simulink model "dmpc"  (R2021a)
settings: Solver=ode4  StartTime=0.0  StopTime=10  FixedStep=simTs  RelTol=1e-3
values from neighbouring files (symbols this model uses):
  simTs = 1e-6    (= 1e-06)    [model.m]
  Ts = 80e-3    (= 0.08)    [model.m]
libraries: pid_lib x9, spsThreePhaseSeriesRLCBranchLib x9, spsabctodq0Lib x9, spsRMSLib x6, spsThreePhaseVIMeasurementLib x6, spsFirstOrderFilterLib x6, spsSecondOrderFilterLib x6, spsThreePhaseSeriesRLCLoadLib x4, spsFourierLib x3, spsPWMGenerator2LevelLib x3, spsdq0toabcLib x3, spsCurrentMeasurementLib x3
(part 1 of 2)
settings Model: SimulationMode=accelerator  Creator=Sameer Kumar  LastModifiedBy=Sameer Kumar

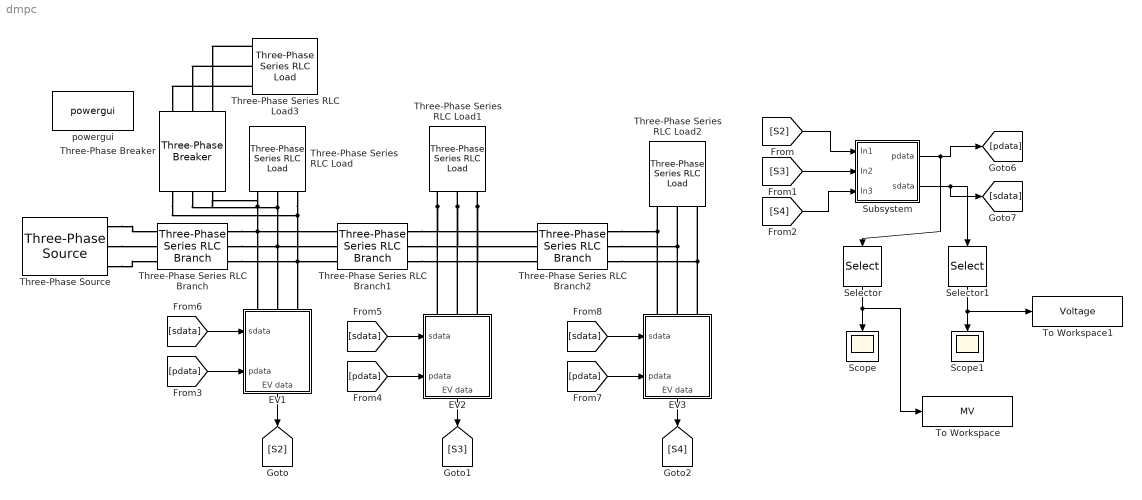
== system dmpc ==
  EV1 : Subsystem
      settings: PortSchema="{\"entries\":[{\"content\":{\"sides\":[{\"content\":{\"connectorIds\":[\"LConn1\",\"LConn2\",\"LConn3\"]},\"type\":\"ConnectorPlacement.EquallySpacedRectSide\",\"uuid\":\"b1121362-91a5-4336-a6ad-67b3009c2f66\"},{\"content\":{\"connectorIds\":[\"Out1\"],\"side\":\"RIGHT\"},\"type\":\"ConnectorPlacement.EquallySpacedRectSide\",\"uuid\":\"ba666203-56ee-4aa1-80fa-3bec4e81a32f\"},{\"content\":{\"connectorIds\":[\"In1\",\"In2\"],\"side\":\"TOP\"},\"type\":\"ConnectorPlacement.EquallySpacedRectSide\",\"uuid\":\"ec91c225-dc43-4f31-ad74-0ab1fa7bfdf2\"}]},\"type\":\"ConnectorPlacement.EquallySpacedConnector\",\"uuid\":\"9ad0d362-2acd-4c24-addb-fb01ea261cc5\"}],\"packageUris\":[\"http://schema.mathworks.com/mf0/Connector/R2020b\"],\"version\":\"1.0\"}"
  EV2 : Subsystem
      settings: PortSchema="{\"entries\":[{\"content\":{\"sides\":[{\"content\":{\"connectorIds\":[\"LConn1\",\"LConn2\",\"LConn3\"]},\"type\":\"ConnectorPlacement.EquallySpacedRectSide\",\"uuid\":\"b1121362-91a5-4336-a6ad-67b3009c2f66\"},{\"content\":{\"connectorIds\":[\"Out1\"],\"side\":\"RIGHT\"},\"type\":\"ConnectorPlacement.EquallySpacedRectSide\",\"uuid\":\"ba666203-56ee-4aa1-80fa-3bec4e81a32f\"},{\"content\":{\"connectorIds\":[\"In1\",\"In2\"],\"side\":\"TOP\"},\"type\":\"ConnectorPlacement.EquallySpacedRectSide\",\"uuid\":\"ec91c225-dc43-4f31-ad74-0ab1fa7bfdf2\"}]},\"type\":\"ConnectorPlacement.EquallySpacedConnector\",\"uuid\":\"9ad0d362-2acd-4c24-addb-fb01ea261cc5\"}],\"packageUris\":[\"http://schema.mathworks.com/mf0/Connector/R2020b\"],\"version\":\"1.0\"}"
  EV3 : Subsystem
      settings: PortSchema="{\"entries\":[{\"content\":{\"sides\":[{\"content\":{\"connectorIds\":[\"LConn1\",\"LConn2\",\"LConn3\"]},\"type\":\"ConnectorPlacement.EquallySpacedRectSide\",\"uuid\":\"b1121362-91a5-4336-a6ad-67b3009c2f66\"},{\"content\":{\"connectorIds\":[\"Out1\"],\"side\":\"RIGHT\"},\"type\":\"ConnectorPlacement.EquallySpacedRectSide\",\"uuid\":\"ba666203-56ee-4aa1-80fa-3bec4e81a32f\"},{\"content\":{\"connectorIds\":[\"In1\",\"In2\"],\"side\":\"TOP\"},\"type\":\"ConnectorPlacement.EquallySpacedRectSide\",\"uuid\":\"ec91c225-dc43-4f31-ad74-0ab1fa7bfdf2\"}]},\"type\":\"ConnectorPlacement.EquallySpacedConnector\",\"uuid\":\"9ad0d362-2acd-4c24-addb-fb01ea261cc5\"}],\"packageUris\":[\"http://schema.mathworks.com/mf0/Connector/R2020b\"],\"version\":\"1.0\"}"
  Scope : Scope
  Scope1 : Scope
  Selector : Selector  InputPortWidth=24  IndexOptions=Index vector (dialog)  Indices=[1 9 17]  OutputSizes=1
  Selector1 : Selector  InputPortWidth=8  IndexOptions=Index vector (dialog)  Indices=[6 7 8]  OutputSizes=1
  Subsystem : Subsystem
  Three-Phase Series RLC Branch : spsThreePhaseSeriesRLCBranchLib/Three-Phase Series RLC Branch  LConnTagsString=A|B|C  RConnTagsString=A|B|C  BranchType=RL  Resistance=0.05  Inductance=0.75e-3  Capacitance=1e-6  Measurements=None
  Three-Phase Series RLC Branch1 : spsThreePhaseSeriesRLCBranchLib/Three-Phase Series RLC Branch  LConnTagsString=A|B|C  RConnTagsString=A|B|C  BranchType=RL  Resistance=0.05  Inductance=0.15e-3  Capacitance=1e-6  Measurements=None
  Three-Phase Series RLC Branch2 : spsThreePhaseSeriesRLCBranchLib/Three-Phase Series RLC Branch  LConnTagsString=A|B|C  RConnTagsString=A|B|C  BranchType=RL  Resistance=0.05  Inductance=0.15e-3  Capacitance=1e-6  Measurements=None
  Three-Phase Series RLC Load : spsThreePhaseSeriesRLCLoadLib/Three-Phase Series RLC Load  LConnTagsString=A|B|C  Configuration=Y (grounded)  NominalVoltage=400  Vabc=[1e3 1e3 1e3]  Vabcp=[1e3 1e3 1e3]  NominalFrequency=50  UnbalancedPower=off  ActivePower=5e3  InductivePower=1.5e3  CapacitivePower=0  Pabc=[10e3 9e3 11e3]  QLabc=[100 90 110]  QCabc=[100 90 110]  Pabcp=[10e3 9e3 11e3]  QLabcp=[100 90 110]  QCabcp=[100 90 110]  Measurements=None  LoadType=constant Z
  Three-Phase Series RLC Load1 : spsThreePhaseSeriesRLCLoadLib/Three-Phase Series RLC Load  LConnTagsString=A|B|C  Configuration=Y (grounded)  NominalVoltage=400  Vabc=[1e3 1e3 1e3]  Vabcp=[1e3 1e3 1e3]  NominalFrequency=50  UnbalancedPower=off  ActivePower=5e3  InductivePower=1e3  CapacitivePower=0  Pabc=[10e3 9e3 11e3]  QLabc=[100 90 110]  QCabc=[100 90 110]  Pabcp=[10e3 9e3 11e3]  QLabcp=[100 90 110]  QCabcp=[100 90 110]  Measurements=None  LoadType=constant Z
  Three-Phase Series RLC Load2 : spsThreePhaseSeriesRLCLoadLib/Three-Phase Series RLC Load  LConnTagsString=A|B|C  Configuration=Y (grounded)  NominalVoltage=400  Vabc=[1e3 1e3 1e3]  Vabcp=[1e3 1e3 1e3]  NominalFrequency=50  UnbalancedPower=off  ActivePower=5e3  InductivePower=1e3  CapacitivePower=0  Pabc=[10e3 9e3 11e3]  QLabc=[100 90 110]  QCabc=[100 90 110]  Pabcp=[10e3 9e3 11e3]  QLabcp=[100 90 110]  QCabcp=[100 90 110]  Measurements=None  LoadType=constant Z
  Three-Phase Series RLC Load3 : spsThreePhaseSeriesRLCLoadLib/Three-Phase Series RLC Load  LConnTagsString=A|B|C  Configuration=Y (grounded)  NominalVoltage=400  Vabc=[1e3 1e3 1e3]  Vabcp=[1e3 1e3 1e3]  NominalFrequency=50  UnbalancedPower=off  ActivePower=0.1e-3  InductivePower=1.5e3  CapacitivePower=0  Pabc=[10e3 9e3 11e3]  QLabc=[100 90 110]  QCabc=[100 90 110]  Pabcp=[10e3 9e3 11e3]  QLabcp=[100 90 110]  QCabcp=[100 90 110]  Measurements=None  LoadType=constant Z
  Three-Phase Breaker : spsThreePhaseBreakerLib/Three-Phase Breaker  InitialState=open  SwitchA=on  SwitchB=on  SwitchC=on  SwitchTimes=[4]  External=off  BreakerResistance=1e-5  SnubberResistance=1e6  SnubberCapacitance=inf  Measurements=None
  Three-Phase Source : spsThreePhaseSourceLib/Three-Phase Source  InternalConnection=Yg  VoltagePhases=off  Voltage=400  PhaseAngle=0  Voltage_phases=[25e3 25e3 25e3]/sqrt(3)  PhaseAngles_phases=[0 -120 +120]  Frequency=50  NonIdealSource=on  SpecifyImpedance=off  Resistance=0  Inductance=0  ShortCircuitLevel=100e6  BaseVoltage=400  XRratio=7  BusType=swing  Pref=10e3  Qref=0  Prefabc=[10e3, 10e3, 10e3]  Qrefabc=[0, 0, 0]  Qmin=-inf  Qmax=inf
  To Workspace : ToWorkspace  VariableName=MV  SaveFormat=Timeseries  SampleTime=-1
  To Workspace1 : ToWorkspace  VariableName=Voltage  SaveFormat=Timeseries  SampleTime=-1
  powergui : spspowerguiLib/powergui  Priority=1  SimulationMode=Discrete  SampleTime=simTs  frequency=60  Iterations=50  frequencyindice=0  Pbase=100e6  ErrMax=1e-4  UnitsV=kV  UnitsW=MW  buscounter=0  FunctionMessages=off  echomessages=off  EnableUseOfTLC=off  CurrentSourceSwitches=off  DisableSnubberDevices=off  DisableRonSwitches=off  DisableVfSwitches=off  DisplayEquations=off  AutomaticDiscreteSolvers=off  SolverType=Tustin/Backward Euler (TBE)  Interpol=off  ExternalGateDelay=off  methode=off  Ts=100  x0status=blocks  SPID=on  SwTol=0  HookPort=off  NonlinearTolerance=1e-4  nMaxIteration=100  ContinueOnMaxIteration=off  RestoreLinks=warning  ResistiveCurrentMeasurement=off  Frange=[0:2:500]  Ylog=off  Xlog=on  ShowGrid=off  save=off  variable=ZData  structure=0  ZoomFFT=off  StartTime=0.0  cycles=1  DisplayStyle=1  fundamental=60  FreqAxis=off  MaxFrequency=1000  frequencyindicesteady=1  RmsSteady=1  display=off
  wires:
  [sdata] -> EV1/1(sdata)
  EV1/1(EV data) -> [S2]
  [pdata] -> EV1/2(pdata)
  [pdata] -> EV2/2(pdata)
  EV2/1(EV data) -> [S3]
  [sdata] -> EV2/1(sdata)
  [pdata] -> EV3/2(pdata)
  EV3/1(EV data) -> [S4]
  [sdata] -> EV3/1(sdata)
  [S2] -> Subsystem/1(In1)
  [S3] -> Subsystem/2(In2)
  [S4] -> Subsystem/3(In3)
  Subsystem/1(pdata) -> [pdata], Selector/1
  Subsystem/2(sdata) -> Selector1/1, [sdata]
  Selector/1 -> To Workspace/1, Scope/1
  Selector1/1 -> To Workspace1/1, Scope1/1
  connections:
  Three-Phase Series RLC Branch2/RConn3 -- EV3/LConn3 -- Three-Phase Series RLC Load2/LConn3
  Three-Phase Series RLC Load1/LConn3 -- EV2/LConn3 -- Three-Phase Series RLC Branch1/RConn3 -- Three-Phase Series RLC Branch2/LConn3
  Three-Phase Series RLC Branch2/RConn1 -- EV3/LConn1 -- Three-Phase Series RLC Load2/LConn1
  Three-Phase Series RLC Load/LConn1 -- Three-Phase Breaker/RConn1 -- EV1/LConn1 -- Three-Phase Series RLC Branch/RConn1 -- Three-Phase Series RLC Branch1/LConn1
  Three-Phase Series RLC Branch2/RConn2 -- EV3/LConn2 -- Three-Phase Series RLC Load2/LConn2
  Three-Phase Series RLC Load1/LConn2 -- EV2/LConn2 -- Three-Phase Series RLC Branch1/RConn2 -- Three-Phase Series RLC Branch2/LConn2
  Three-Phase Series RLC Load/LConn2 -- Three-Phase Breaker/RConn2 -- EV1/LConn2 -- Three-Phase Series RLC Branch1/LConn2 -- Three-Phase Series RLC Branch/RConn2
  Three-Phase Series RLC Load1/LConn1 -- EV2/LConn1 -- Three-Phase Series RLC Branch1/RConn1 -- Three-Phase Series RLC Branch2/LConn1
  Three-Phase Series RLC Load/LConn3 -- Three-Phase Breaker/RConn3 -- Three-Phase Series RLC Branch1/LConn3 -- EV1/LConn3 -- Three-Phase Series RLC Branch/RConn3
  Three-Phase Source/RConn3 -- Three-Phase Series RLC Branch/LConn3
  Three-Phase Source/RConn1 -- Three-Phase Series RLC Branch/LConn1
  Three-Phase Source/RConn2 -- Three-Phase Series RLC Branch/LConn2
  Three-Phase Series RLC Load3/LConn1 -- Three-Phase Breaker/LConn1
  Three-Phase Series RLC Load3/LConn2 -- Three-Phase Breaker/LConn2
  Three-Phase Series RLC Load3/LConn3 -- Three-Phase Breaker/LConn3

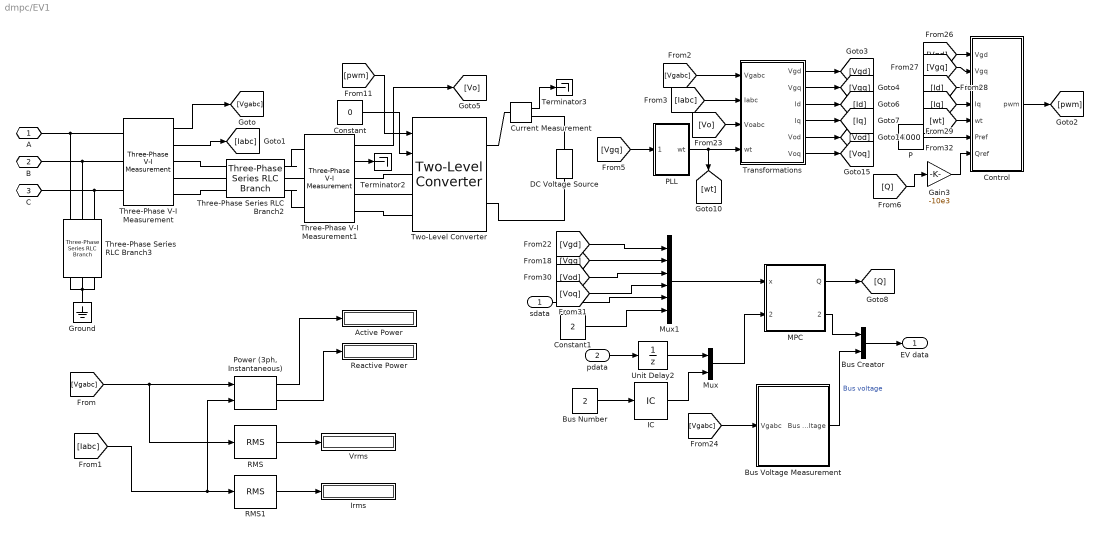
== system dmpc/EV1 ==
  sdata : Inport
  pdata : Inport  Port=2
  Active Power : Display
  Bus Creator : BusCreator  Inputs=2
  Bus Number : Constant  Value=2
  Bus Voltage Measurement : Subsystem
  Constant : Constant  Value=0
  Constant1 : Constant  Value=2
  Control : Subsystem
  Current Measurement : spsCurrentMeasurementLib/Current Measurement  PhasorSimulation=off  OutputType=Complex  PSBequivalent=0
  DC Voltage Source : spsDCVoltageSourceLib/DC Voltage Source  Amplitude=800  Measurements=None
  Gain3 : Gain  Gain=-10e3
  Ground : spsGroundLib/Ground  LConnTagsString=a
  IC : InitialCondition  Value=2
  Irms : Display
  MPC : Subsystem
  Mux : Mux  Inputs=2
  Mux1 : Mux  Inputs=6
  P : Constant  Value=6000
  PLL : Subsystem
  "Power (3ph, Instantaneous)" : spsPower3phInstantaneousLib/Power (3ph, Instantaneous)
  RMS : spsRMSLib/RMS  TrueRMS=on  Freq=50  RMSInit=220  Ts=simTs
  RMS1 : spsRMSLib/RMS  TrueRMS=on  Freq=50  RMSInit=10  Ts=simTs
  Reactive Power : Display
  Terminator2 : Terminator
  Terminator3 : Terminator
  Three-Phase Series RLC Branch2 : spsThreePhaseSeriesRLCBranchLib/Three-Phase Series RLC Branch  LConnTagsString=A|B|C  RConnTagsString=A|B|C  BranchType=RL  Resistance=0.1  Inductance=10e-3  Capacitance=1e-6  Measurements=None
  Three-Phase Series RLC Branch3 : spsThreePhaseSeriesRLCBranchLib/Three-Phase Series RLC Branch  LConnTagsString=A|B|C  RConnTagsString=A|B|C  BranchType=RC  Resistance=1e-3  Inductance=2.5e-3  Capacitance=5e-6  Measurements=None
  Three-Phase V-I Measurement : spsThreePhaseVIMeasurementLib/Three-Phase V-I Measurement  VoltageMeasurement=phase-to-ground  SetLabelV=off  LabelV=Vabc  Vpu=off  VpuLL=off  CurrentMeasurement=yes  SetLabelI=off  LabelI=Iabc  Ipu=off  Pbase=100e6  Vbase=500e3  OutputType=Complex  PhasorSimulation=off  PSBequivalent=0
  Three-Phase V-I Measurement1 : spsThreePhaseVIMeasurementLib/Three-Phase V-I Measurement  VoltageMeasurement=phase-to-ground  SetLabelV=off  LabelV=Vabc  Vpu=off  VpuLL=off  CurrentMeasurement=yes  SetLabelI=off  LabelI=Iabc  Ipu=off  Pbase=100e6  Vbase=500e3  OutputType=Complex  PhasorSimulation=off  PSBequivalent=0
  Transformations : Subsystem
  Two-Level Converter : spsTwoLevelConverterLib/Two-Level Converter  ModelType=Switching devices  Ron=1e-3  Rs=1e6  Cs=inf  Vforward=[0,0]  Ron_Diode=1e-3  Rs_Diode=1e6  Cs_Diode=inf  Vf_Diode=1e-3  Rs_CurrentSource=inf
      settings: SourceProductBaseCode=PS
  Unit Delay2 : UnitDelay  SampleTime=simTs  HasFrameUpgradeWarning=on
  Vrms : Display
  A : PMIOPort  Side=Left
  B : PMIOPort  Port=2  Side=Left
  C : PMIOPort  Port=3  Side=Left
  EV data : Outport
  wires:
  [pwm] -> Two-Level Converter/1
  Current Measurement/1 -> Terminator3/1
  Three-Phase V-I Measurement/1 -> [Vgabc]
  Three-Phase V-I Measurement/2 -> [Iabc]
  [Vgabc] -> Transformations/1(Vgabc)
  [Iabc] -> Transformations/2(Iabc)
  Transformations/1(Vgd) -> [Vgd]
  Transformations/2(Vgq) -> [Vgq]
  Transformations/3(Id) -> [Id]
  Transformations/4(Iq) -> [Iq]
  PLL/1(wt) -> Transformations/4(wt), [wt]
  [Vgq] -> PLL/1(Vgq)
  Control/1(pwm) -> [pwm]
  Three-Phase V-I Measurement1/1 -> [Vo]
  [Vo] -> Transformations/3(Voabc)
  Transformations/5(Vod) -> [Vod]
  Transformations/6(Voq) -> [Voq]
  [wt] -> Control/5(wt)
  [Vgd] -> Control/1(Vgd)
  [Vgq] -> Control/2(Vgq)
  [Id] -> Control/3(Id)
  [Iq] -> Control/4(Iq)
  P/1 -> Control/6(Pref)
  RMS/1 -> Vrms/1
  "Power (3ph, Instantaneous)"/1 -> Active Power/1
  "Power (3ph, Instantaneous)"/2 -> Reactive Power/1
  [Vgabc] -> "Power (3ph, Instantaneous)"/1, RMS/1
  [Iabc] -> "Power (3ph, Instantaneous)"/2, RMS1/1
  RMS1/1 -> Irms/1
  [Q] -> Gain3/1
  Gain3/1 -> Control/7(Qref)
  Constant/1 -> Two-Level Converter/2
  Three-Phase V-I Measurement1/2 -> Terminator2/1
  Mux1/1 -> MPC/1(x)
  MPC/1(Q) -> [Q]
  [Vgd] -> Mux1/1
  [Vgq] -> Mux1/2
  [Vod] -> Mux1/3
  [Voq] -> Mux1/4
  Bus Voltage Measurement/1(Bus Voltage) -> Bus Creator/2  "Bus voltage"
  [Vgabc] -> Bus Voltage Measurement/1(Vgabc)
  MPC/2(mvpred) -> Bus Creator/1
  Bus Creator/1 -> EV data/1
  Constant1/1 -> Mux1/6
  sdata/1 -> Mux1/5
  Mux/1 -> MPC/2(params)
  Bus Number/1 -> IC/1
  IC/1 -> Mux/2
  pdata/1 -> Unit Delay2/1
  Unit Delay2/1 -> Mux/1
  connections:
  Current Measurement/RConn1 -- DC Voltage Source/RConn1
  Two-Level Converter/RConn2 -- DC Voltage Source/LConn1
  Two-Level Converter/RConn1 -- Current Measurement/LConn1
  A/RConn1 -- Three-Phase Series RLC Branch3/LConn1 -- Three-Phase V-I Measurement/LConn1
  B/RConn1 -- Three-Phase Series RLC Branch3/LConn2 -- Three-Phase V-I Measurement/LConn2
  C/RConn1 -- Three-Phase Series RLC Branch3/LConn3 -- Three-Phase V-I Measurement/LConn3
  Two-Level Converter/LConn1 -- Three-Phase V-I Measurement1/RConn1
  Two-Level Converter/LConn2 -- Three-Phase V-I Measurement1/RConn2
  Two-Level Converter/LConn3 -- Three-Phase V-I Measurement1/RConn3
  Ground/LConn1 -- Three-Phase Series RLC Branch3/RConn3 -- Three-Phase Series RLC Branch3/RConn2 -- Three-Phase Series RLC Branch3/RConn1
  Three-Phase Series RLC Branch2/RConn1 -- Three-Phase V-I Measurement1/LConn1
  Three-Phase Series RLC Branch2/RConn2 -- Three-Phase V-I Measurement1/LConn2
  Three-Phase Series RLC Branch2/RConn3 -- Three-Phase V-I Measurement1/LConn3
  Three-Phase V-I Measurement/RConn1 -- Three-Phase Series RLC Branch2/LConn1
  Three-Phase V-I Measurement/RConn2 -- Three-Phase Series RLC Branch2/LConn2
  Three-Phase V-I Measurement/RConn3 -- Three-Phase Series RLC Branch2/LConn3

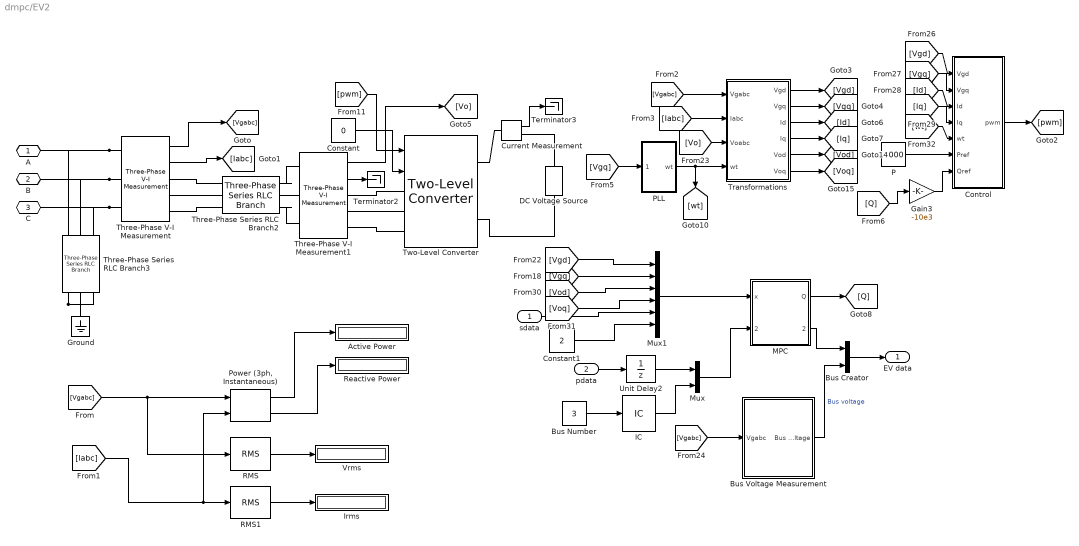
== system dmpc/EV2 ==
  sdata : Inport
  pdata : Inport  Port=2
  Active Power : Display
  Bus Creator : BusCreator  Inputs=2
  Bus Number : Constant  Value=3
  Bus Voltage Measurement : Subsystem
  Constant : Constant  Value=0
  Constant1 : Constant  Value=2
  Control : Subsystem
  Current Measurement : spsCurrentMeasurementLib/Current Measurement  PhasorSimulation=off  OutputType=Complex  PSBequivalent=0
  DC Voltage Source : spsDCVoltageSourceLib/DC Voltage Source  Amplitude=800  Measurements=None
  Gain3 : Gain  Gain=-10e3
  Ground : spsGroundLib/Ground  LConnTagsString=a
  IC : InitialCondition  Value=3
  Irms : Display
  MPC : Subsystem
  Mux : Mux  Inputs=2
  Mux1 : Mux  Inputs=6
  P : Constant  Value=6000
  PLL : Subsystem
  "Power (3ph, Instantaneous)" : spsPower3phInstantaneousLib/Power (3ph, Instantaneous)
  RMS : spsRMSLib/RMS  TrueRMS=on  Freq=50  RMSInit=220  Ts=simTs
  RMS1 : spsRMSLib/RMS  TrueRMS=on  Freq=50  RMSInit=10  Ts=simTs
  Reactive Power : Display
  Terminator2 : Terminator
  Terminator3 : Terminator
  Three-Phase Series RLC Branch2 : spsThreePhaseSeriesRLCBranchLib/Three-Phase Series RLC Branch  LConnTagsString=A|B|C  RConnTagsString=A|B|C  BranchType=RL  Resistance=0.1  Inductance=10e-3  Capacitance=1e-6  Measurements=None
  Three-Phase Series RLC Branch3 : spsThreePhaseSeriesRLCBranchLib/Three-Phase Series RLC Branch  LConnTagsString=A|B|C  RConnTagsString=A|B|C  BranchType=RC  Resistance=1e-3  Inductance=2.5e-3  Capacitance=5e-6  Measurements=None
  Three-Phase V-I Measurement : spsThreePhaseVIMeasurementLib/Three-Phase V-I Measurement  VoltageMeasurement=phase-to-ground  SetLabelV=off  LabelV=Vabc  Vpu=off  VpuLL=off  CurrentMeasurement=yes  SetLabelI=off  LabelI=Iabc  Ipu=off  Pbase=100e6  Vbase=500e3  OutputType=Complex  PhasorSimulation=off  PSBequivalent=0
  Three-Phase V-I Measurement1 : spsThreePhaseVIMeasurementLib/Three-Phase V-I Measurement  VoltageMeasurement=phase-to-ground  SetLabelV=off  LabelV=Vabc  Vpu=off  VpuLL=off  CurrentMeasurement=yes  SetLabelI=off  LabelI=Iabc  Ipu=off  Pbase=100e6  Vbase=500e3  OutputType=Complex  PhasorSimulation=off  PSBequivalent=0
  Transformations : Subsystem
  Two-Level Converter : spsTwoLevelConverterLib/Two-Level Converter  ModelType=Switching devices  Ron=1e-3  Rs=1e6  Cs=inf  Vforward=[0,0]  Ron_Diode=1e-3  Rs_Diode=1e6  Cs_Diode=inf  Vf_Diode=1e-3  Rs_CurrentSource=inf
      settings: SourceProductBaseCode=PS
  Unit Delay2 : UnitDelay  SampleTime=simTs  HasFrameUpgradeWarning=on
  Vrms : Display
  A : PMIOPort  Side=Left
  B : PMIOPort  Port=2  Side=Left
  C : PMIOPort  Port=3  Side=Left
  EV data : Outport
  wires:
  Unit Delay2/1 -> Mux/1
  pdata/1 -> Unit Delay2/1
  IC/1 -> Mux/2
  Bus Number/1 -> IC/1
  Mux/1 -> MPC/2(params)
  sdata/1 -> Mux1/5
  Constant1/1 -> Mux1/6
  Bus Creator/1 -> EV data/1
  MPC/2(mvpred) -> Bus Creator/1
  [Vgabc] -> Bus Voltage Measurement/1(Vgabc)
  Bus Voltage Measurement/1(Bus Voltage) -> Bus Creator/2  "Bus voltage"
  [Voq] -> Mux1/4
  [Vod] -> Mux1/3
  [Vgq] -> Mux1/2
  [Vgd] -> Mux1/1
  MPC/1(Q) -> [Q]
  Mux1/1 -> MPC/1(x)
  Three-Phase V-I Measurement1/2 -> Terminator2/1
  Constant/1 -> Two-Level Converter/2
  Gain3/1 -> Control/7(Qref)
  [Q] -> Gain3/1
  RMS1/1 -> Irms/1
  [Iabc] -> RMS1/1, "Power (3ph, Instantaneous)"/2
  [Vgabc] -> RMS/1, "Power (3ph, Instantaneous)"/1
  "Power (3ph, Instantaneous)"/2 -> Reactive Power/1
  "Power (3ph, Instantaneous)"/1 -> Active Power/1
  RMS/1 -> Vrms/1
  P/1 -> Control/6(Pref)
  [Iq] -> Control/4(Iq)
  [Id] -> Control/3(Id)
  [Vgq] -> Control/2(Vgq)
  [Vgd] -> Control/1(Vgd)
  [wt] -> Control/5(wt)
  Transformations/6(Voq) -> [Voq]
  Transformations/5(Vod) -> [Vod]
  [Vo] -> Transformations/3(Voabc)
  Three-Phase V-I Measurement1/1 -> [Vo]
  Control/1(pwm) -> [pwm]
  [Vgq] -> PLL/1(Vgq)
  PLL/1(wt) -> [wt], Transformations/4(wt)
  Transformations/4(Iq) -> [Iq]
  Transformations/3(Id) -> [Id]
  Transformations/2(Vgq) -> [Vgq]
  Transformations/1(Vgd) -> [Vgd]
  [Iabc] -> Transformations/2(Iabc)
  [Vgabc] -> Transformations/1(Vgabc)
  Three-Phase V-I Measurement/2 -> [Iabc]
  Three-Phase V-I Measurement/1 -> [Vgabc]
  Current Measurement/1 -> Terminator3/1
  [pwm] -> Two-Level Converter/1
  connections:
  Three-Phase V-I Measurement/RConn3 -- Three-Phase Series RLC Branch2/LConn3
  Three-Phase V-I Measurement/RConn2 -- Three-Phase Series RLC Branch2/LConn2
  Three-Phase V-I Measurement/RConn1 -- Three-Phase Series RLC Branch2/LConn1
  Three-Phase Series RLC Branch2/RConn3 -- Three-Phase V-I Measurement1/LConn3
  Three-Phase Series RLC Branch2/RConn2 -- Three-Phase V-I Measurement1/LConn2
  Three-Phase Series RLC Branch2/RConn1 -- Three-Phase V-I Measurement1/LConn1
  Three-Phase Series RLC Branch3/RConn1 -- Three-Phase Series RLC Branch3/RConn2 -- Three-Phase Series RLC Branch3/RConn3 -- Ground/LConn1
  Two-Level Converter/LConn3 -- Three-Phase V-I Measurement1/RConn3
  Two-Level Converter/LConn2 -- Three-Phase V-I Measurement1/RConn2
  Two-Level Converter/LConn1 -- Three-Phase V-I Measurement1/RConn1
  Three-Phase V-I Measurement/LConn3 -- Three-Phase Series RLC Branch3/LConn3 -- C/RConn1
  Three-Phase V-I Measurement/LConn2 -- Three-Phase Series RLC Branch3/LConn2 -- B/RConn1
  Three-Phase V-I Measurement/LConn1 -- Three-Phase Series RLC Branch3/LConn1 -- A/RConn1
  Two-Level Converter/RConn1 -- Current Measurement/LConn1
  Two-Level Converter/RConn2 -- DC Voltage Source/LConn1
  Current Measurement/RConn1 -- DC Voltage Source/RConn1

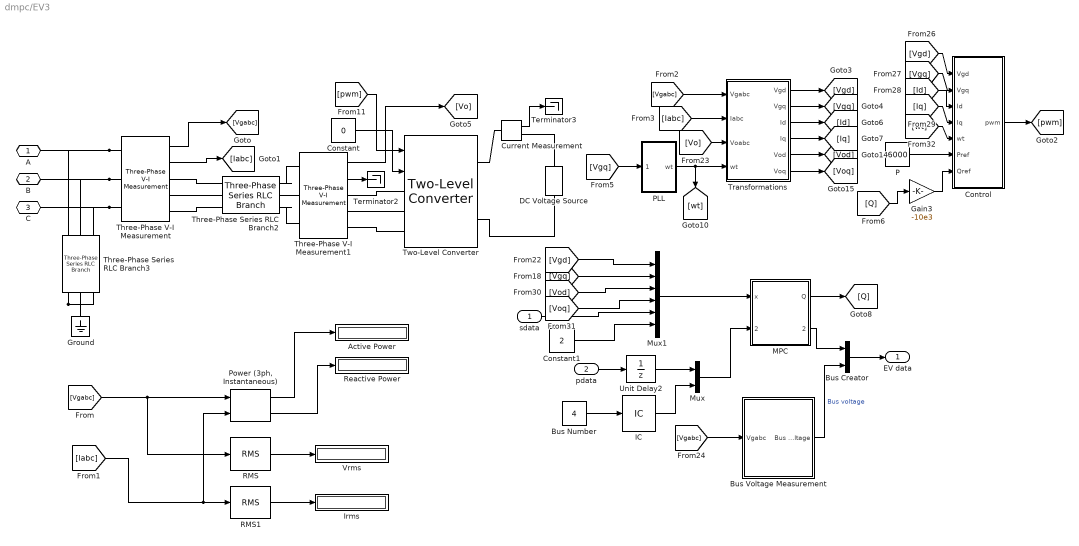
== system dmpc/EV3 ==
  sdata : Inport
  pdata : Inport  Port=2
  Active Power : Display
  Bus Creator : BusCreator  Inputs=2
  Bus Number : Constant  Value=4
  Bus Voltage Measurement : Subsystem
  Constant : Constant  Value=0
  Constant1 : Constant  Value=2
  Control : Subsystem
  Current Measurement : spsCurrentMeasurementLib/Current Measurement  PhasorSimulation=off  OutputType=Complex  PSBequivalent=0
  DC Voltage Source : spsDCVoltageSourceLib/DC Voltage Source  Amplitude=800  Measurements=None
  Gain3 : Gain  Gain=-10e3
  Ground : spsGroundLib/Ground  LConnTagsString=a
  IC : InitialCondition  Value=4
  Irms : Display
  MPC : Subsystem
  Mux : Mux  Inputs=2
  Mux1 : Mux  Inputs=6
  P : Constant  Value=6000
  PLL : Subsystem
  "Power (3ph, Instantaneous)" : spsPower3phInstantaneousLib/Power (3ph, Instantaneous)
  RMS : spsRMSLib/RMS  TrueRMS=on  Freq=50  RMSInit=220  Ts=simTs
  RMS1 : spsRMSLib/RMS  TrueRMS=on  Freq=50  RMSInit=10  Ts=simTs
  Reactive Power : Display
  Terminator2 : Terminator
  Terminator3 : Terminator
  Three-Phase Series RLC Branch2 : spsThreePhaseSeriesRLCBranchLib/Three-Phase Series RLC Branch  LConnTagsString=A|B|C  RConnTagsString=A|B|C  BranchType=RL  Resistance=0.1  Inductance=10e-3  Capacitance=1e-6  Measurements=None
  Three-Phase Series RLC Branch3 : spsThreePhaseSeriesRLCBranchLib/Three-Phase Series RLC Branch  LConnTagsString=A|B|C  RConnTagsString=A|B|C  BranchType=RC  Resistance=1e-3  Inductance=2.5e-3  Capacitance=5e-6  Measurements=None
  Three-Phase V-I Measurement : spsThreePhaseVIMeasurementLib/Three-Phase V-I Measurement  VoltageMeasurement=phase-to-ground  SetLabelV=off  LabelV=Vabc  Vpu=off  VpuLL=off  CurrentMeasurement=yes  SetLabelI=off  LabelI=Iabc  Ipu=off  Pbase=100e6  Vbase=500e3  OutputType=Complex  PhasorSimulation=off  PSBequivalent=0
  Three-Phase V-I Measurement1 : spsThreePhaseVIMeasurementLib/Three-Phase V-I Measurement  VoltageMeasurement=phase-to-ground  SetLabelV=off  LabelV=Vabc  Vpu=off  VpuLL=off  CurrentMeasurement=yes  SetLabelI=off  LabelI=Iabc  Ipu=off  Pbase=100e6  Vbase=500e3  OutputType=Complex  PhasorSimulation=off  PSBequivalent=0
  Transformations : Subsystem
  Two-Level Converter : spsTwoLevelConverterLib/Two-Level Converter  ModelType=Switching devices  Ron=1e-3  Rs=1e6  Cs=inf  Vforward=[0,0]  Ron_Diode=1e-3  Rs_Diode=1e6  Cs_Diode=inf  Vf_Diode=1e-3  Rs_CurrentSource=inf
      settings: SourceProductBaseCode=PS
  Unit Delay2 : UnitDelay  SampleTime=simTs  HasFrameUpgradeWarning=on
  Vrms : Display
  A : PMIOPort  Side=Left
  B : PMIOPort  Port=2  Side=Left
  C : PMIOPort  Port=3  Side=Left
  EV data : Outport
  wires:
  Unit Delay2/1 -> Mux/1
  pdata/1 -> Unit Delay2/1
  IC/1 -> Mux/2
  Bus Number/1 -> IC/1
  Mux/1 -> MPC/2(params)
  sdata/1 -> Mux1/5
  Constant1/1 -> Mux1/6
  Bus Creator/1 -> EV data/1
  MPC/2(mvpred) -> Bus Creator/1
  [Vgabc] -> Bus Voltage Measurement/1(Vgabc)
  Bus Voltage Measurement/1(Bus Voltage) -> Bus Creator/2  "Bus voltage"
  [Voq] -> Mux1/4
  [Vod] -> Mux1/3
  [Vgq] -> Mux1/2
  [Vgd] -> Mux1/1
  MPC/1(Q) -> [Q]
  Mux1/1 -> MPC/1(x)
  Three-Phase V-I Measurement1/2 -> Terminator2/1
  Constant/1 -> Two-Level Converter/2
  Gain3/1 -> Control/7(Qref)
  [Q] -> Gain3/1
  RMS1/1 -> Irms/1
  [Iabc] -> RMS1/1, "Power (3ph, Instantaneous)"/2
  [Vgabc] -> RMS/1, "Power (3ph, Instantaneous)"/1
  "Power (3ph, Instantaneous)"/2 -> Reactive Power/1
  "Power (3ph, Instantaneous)"/1 -> Active Power/1
  RMS/1 -> Vrms/1
  P/1 -> Control/6(Pref)
  [Iq] -> Control/4(Iq)
  [Id] -> Control/3(Id)
  [Vgq] -> Control/2(Vgq)
  [Vgd] -> Control/1(Vgd)
  [wt] -> Control/5(wt)
  Transformations/6(Voq) -> [Voq]
  Transformations/5(Vod) -> [Vod]
  [Vo] -> Transformations/3(Voabc)
  Three-Phase V-I Measurement1/1 -> [Vo]
  Control/1(pwm) -> [pwm]
  [Vgq] -> PLL/1(Vgq)
  PLL/1(wt) -> [wt], Transformations/4(wt)
  Transformations/4(Iq) -> [Iq]
  Transformations/3(Id) -> [Id]
  Transformations/2(Vgq) -> [Vgq]
  Transformations/1(Vgd) -> [Vgd]
  [Iabc] -> Transformations/2(Iabc)
  [Vgabc] -> Transformations/1(Vgabc)
  Three-Phase V-I Measurement/2 -> [Iabc]
  Three-Phase V-I Measurement/1 -> [Vgabc]
  Current Measurement/1 -> Terminator3/1
  [pwm] -> Two-Level Converter/1
  connections:
  Three-Phase V-I Measurement/RConn3 -- Three-Phase Series RLC Branch2/LConn3
  Three-Phase V-I Measurement/RConn2 -- Three-Phase Series RLC Branch2/LConn2
  Three-Phase V-I Measurement/RConn1 -- Three-Phase Series RLC Branch2/LConn1
  Three-Phase Series RLC Branch2/RConn3 -- Three-Phase V-I Measurement1/LConn3
  Three-Phase Series RLC Branch2/RConn2 -- Three-Phase V-I Measurement1/LConn2
  Three-Phase Series RLC Branch2/RConn1 -- Three-Phase V-I Measurement1/LConn1
  Three-Phase Series RLC Branch3/RConn1 -- Three-Phase Series RLC Branch3/RConn2 -- Three-Phase Series RLC Branch3/RConn3 -- Ground/LConn1
  Two-Level Converter/LConn3 -- Three-Phase V-I Measurement1/RConn3
  Two-Level Converter/LConn2 -- Three-Phase V-I Measurement1/RConn2
  Two-Level Converter/LConn1 -- Three-Phase V-I Measurement1/RConn1
  Three-Phase V-I Measurement/LConn3 -- Three-Phase Series RLC Branch3/LConn3 -- C/RConn1
  Three-Phase V-I Measurement/LConn2 -- Three-Phase Series RLC Branch3/LConn2 -- B/RConn1
  Three-Phase V-I Measurement/LConn1 -- Three-Phase Series RLC Branch3/LConn1 -- A/RConn1
  Two-Level Converter/RConn1 -- Current Measurement/LConn1
  Two-Level Converter/RConn2 -- DC Voltage Source/LConn1
  Current Measurement/RConn1 -- DC Voltage Source/RConn1

== system dmpc/Subsystem ==
  In1 : Inport
  In2 : Inport  Port=2
  In3 : Inport  Port=3
  Bus Creator : BusCreator  Inputs=5
  Bus Selector : BusSelector  OutputSignals=Bus2.mvpred,Bus3.mvpred,Bus4.mvpred,signal4,Bus2.Bus voltage.theta,Bus3.Bus voltage.theta,Bus4.Bus voltage.theta,signal5,Bus2.Bus voltage.voltage,Bus3.Bus voltage.voltage,Bus4.Bus voltage.voltage
  Constant : Constant  Value=0
  Constant1 : Constant
  Mux : Mux  Inputs=3
  Mux1 : Mux  Inputs=8
  pdata : Outport
  sdata : Outport  Port=2
  wires:
  In3/1 -> Bus Creator/3  "Bus4"
  In2/1 -> Bus Creator/2  "Bus3"
  In1/1 -> Bus Creator/1  "Bus2"
  Constant/1 -> Bus Creator/4
  Constant1/1 -> Bus Creator/5
  Bus Selector/1 -> Mux/1  "<mvpred>"
  Bus Selector/2 -> Mux/2  "<mvpred>"
  Bus Selector/3 -> Mux/3  "<mvpred>"
  Mux/1 -> pdata/1
  Bus Selector/4 -> Mux1/1  "<signal4>"
  Bus Selector/5 -> Mux1/2  "<theta>"
  Bus Selector/6 -> Mux1/3  "<theta>"
  Bus Selector/7 -> Mux1/4  "<theta>"
  Bus Selector/8 -> Mux1/5  "<signal5>"
  Bus Selector/9 -> Mux1/6  "<voltage>"
  Bus Selector/10 -> Mux1/7  "<voltage>"
  Bus Selector/11 -> Mux1/8  "<voltage>"
  Mux1/1 -> sdata/1
  Bus Creator/1 -> Bus Selector/1

== system dmpc/EV1/Bus Voltage Measurement ==
  Vgabc : Inport
  Bus Creator : BusCreator  Inputs=2
  Demux : Demux  Outputs=3
  Fourier1 : spsFourierLib/Fourier  Freq=50  n=1  InInit=[300, 0]  Ts=simTs
      settings: SourceProductBaseCode=PS
  Gain : Gain  Gain=sqrt(3/2)/400
  Gain1 : Gain  Gain=pi/180
  Scope : Scope
  Terminator : Terminator
  Terminator1 : Terminator
  Bus Voltage : Outport
  wires:
  Demux/3 -> Terminator1/1
  Demux/2 -> Terminator/1
  Fourier1/2 -> Gain1/1
  Gain1/1 -> Bus Creator/1, Scope/1  "theta"
  Vgabc/1 -> Demux/1
  Demux/1 -> Fourier1/1
  Fourier1/1 -> Gain/1
  Bus Creator/1 -> Bus Voltage/1
  Gain/1 -> Bus Creator/2  "voltage"

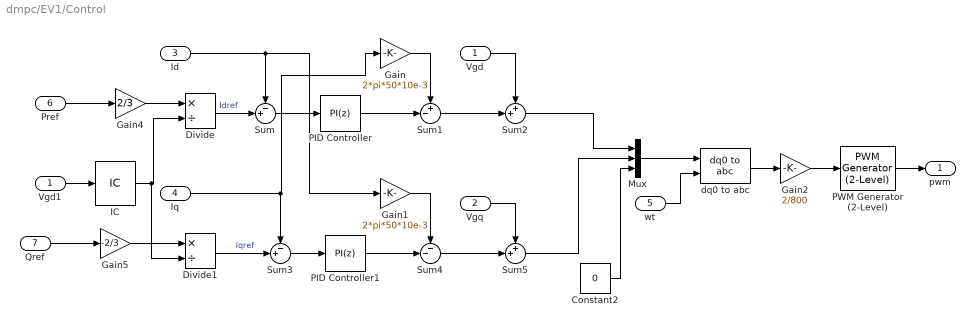
== system dmpc/EV1/Control ==
  Vgd : Inport
  Vgq : Inport  Port=2
  Id : Inport  Port=3
  Iq : Inport  Port=4
  wt : Inport  Port=5
  Pref : Inport  Port=6
  Qref : Inport  Port=7
  Constant2 : Constant  Value=0
  Divide : Product  Inputs=*/
  Divide1 : Product  Inputs=*/
  Gain : Gain  Gain=2*pi*50*10e-3
  Gain1 : Gain  Gain=2*pi*50*10e-3
  Gain2 : Gain  Gain=2/800
  Gain4 : Gain  Gain=2/3
  Gain5 : Gain  Gain=-2/3
  IC : InitialCondition  Value=-300
  Mux : Mux  Inputs=3
  PID Controller : pid_lib/PID Controller  Controller=PI  Form=Parallel  TimeDomain=Discrete-time  UseExternalTs=off  SampleTime=0.1e-3  IntegratorMethod=Forward Euler  FilterMethod=Forward Euler  ControllerParametersSource=internal  P=9  I=2400  D=0  UseFilter=on  N=100  TunerSelectOption=Transfer Function Based (PID Tuner App)  InitialConditionSource=internal  InitialConditionForIntegrator=0  InitialConditionForFilter=0  DifferentiatorICPrevScaledInput=0  ExternalReset=none  TrackingMode=off  Kt=1  LimitOutput=off  SatLimitsSource=internal  UpperSaturationLimit=inf  LowerSaturationLimit=-inf  LinearizeAsGain=on  AntiWindupMode=none  Kb=1  POutMin=[]  POutMax=[]  IOutMin=[]  IOutMax=[]  DOutMin=[]  DOutMax=[]  NOutMin=[]  NOutMax=[]  SumOutMin=[]  SumOutMax=[]  SaturationOutMin=[]  SaturationOutMax=[]  PParamMin=[]  PParamMax=[]  IParamMin=[]  IParamMax=[]  DParamMin=[]  DParamMax=[]  NParamMin=[]  NParamMax=[]  KbParamMin=[]  KbParamMax=[]  KtParamMin=[]  KtParamMax=[]  KbOutMin=[]  KbOutMax=[]  KtOutMin=[]  KtOutMax=[]  IntegratorOutMin=[]  IntegratorOutMax=[]  FilterOutMin=[]  FilterOutMax=[]  SumI1OutMin=[]  SumI1OutMax=[]  SumI2OutMin=[]  SumI2OutMax=[]  SumI3OutMin=[]  SumI3OutMax=[]  SumI4OutMin=[]  SumI4OutMax=[]  SumDOutMin=[]  SumDOutMax=[]  DifferentiatorOutMin=[]  DifferentiatorOutMax=[]  FilterDiffOutCoefMin=[]  FilterDiffOutCoefMax=[]  ReciprocalOutMin=[]  ReciprocalOutMax=[]  SumDenOutMin=[]  SumDenOutMax=[]  SumNumOutMin=[]  SumNumOutMax=[]  DivideOutMin=[]  DivideOutMax=[]  UdiffTsProdOutMin=[]  UdiffTsProdOutMax=[]  NTsProdOutMin=[]  NTsProdOutMax=[]  UintegralTsProdOutMin=[]  UintegralTsProdOutMax=[]  UngainTsProdOutMin=[]  UngainTsProdOutMax=[]  IntegratorContinuousStateAttributes=''  IntegratorStateMustResolveToSignalObject=off  IntegratorRTWStateStorageClass=Auto  FilterContinuousStateAttributes=''  FilterStateMustResolveToSignalObject=off  FilterRTWStateStorageClass=Auto  ParallelPVariant=InternalParameters  IdealPVariant=Disabled  IVariant=InternalParameters  DVariant=Disabled  IntegratorVariant=Discrete  SatVariant=Disabled  AWVariant=Passthrough  PCopyVariant=Disabled  TRVariant=Disabled  FdbkBlocksVariant=Forward  IdealPFdbkVariant=Disabled  SatFdbkVariant=Disabled  DerivativeFilterVariant=Disabled  NVariant=Disabled  NCopyVariant=Disabled_SignalSpec  FilterICVariant=Disabled  IntegratorICVariant=InternalICs  ExternalResetVariant=Disabled  TRSumVariant=Passthrough  SumFdbkVariant=Disabled  SumVariant=Sum_PI  TsampFilterVariant=InternalTs  TsampNgainVariant=Passthrough  TsampIntegralVariant=Passthrough  ExternalSaturationOutDataTypeStr=Inherit: Same as second input
  PID Controller1 : pid_lib/PID Controller  Controller=PI  Form=Parallel  TimeDomain=Discrete-time  UseExternalTs=off  SampleTime=0.1e-3  IntegratorMethod=Forward Euler  FilterMethod=Forward Euler  ControllerParametersSource=internal  P=9  I=2400  D=0  UseFilter=on  N=100  TunerSelectOption=Transfer Function Based (PID Tuner App)  InitialConditionSource=internal  InitialConditionForIntegrator=0  InitialConditionForFilter=0  DifferentiatorICPrevScaledInput=0  ExternalReset=none  TrackingMode=off  Kt=1  LimitOutput=off  SatLimitsSource=internal  UpperSaturationLimit=inf  LowerSaturationLimit=-inf  LinearizeAsGain=on  AntiWindupMode=none  Kb=1  POutMin=[]  POutMax=[]  IOutMin=[]  IOutMax=[]  DOutMin=[]  DOutMax=[]  NOutMin=[]  NOutMax=[]  SumOutMin=[]  SumOutMax=[]  SaturationOutMin=[]  SaturationOutMax=[]  PParamMin=[]  PParamMax=[]  IParamMin=[]  IParamMax=[]  DParamMin=[]  DParamMax=[]  NParamMin=[]  NParamMax=[]  KbParamMin=[]  KbParamMax=[]  KtParamMin=[]  KtParamMax=[]  KbOutMin=[]  KbOutMax=[]  KtOutMin=[]  KtOutMax=[]  IntegratorOutMin=[]  IntegratorOutMax=[]  FilterOutMin=[]  FilterOutMax=[]  SumI1OutMin=[]  SumI1OutMax=[]  SumI2OutMin=[]  SumI2OutMax=[]  SumI3OutMin=[]  SumI3OutMax=[]  SumI4OutMin=[]  SumI4OutMax=[]  SumDOutMin=[]  SumDOutMax=[]  DifferentiatorOutMin=[]  DifferentiatorOutMax=[]  FilterDiffOutCoefMin=[]  FilterDiffOutCoefMax=[]  ReciprocalOutMin=[]  ReciprocalOutMax=[]  SumDenOutMin=[]  SumDenOutMax=[]  SumNumOutMin=[]  SumNumOutMax=[]  DivideOutMin=[]  DivideOutMax=[]  UdiffTsProdOutMin=[]  UdiffTsProdOutMax=[]  NTsProdOutMin=[]  NTsProdOutMax=[]  UintegralTsProdOutMin=[]  UintegralTsProdOutMax=[]  UngainTsProdOutMin=[]  UngainTsProdOutMax=[]  IntegratorContinuousStateAttributes=''  IntegratorStateMustResolveToSignalObject=off  IntegratorRTWStateStorageClass=Auto  FilterContinuousStateAttributes=''  FilterStateMustResolveToSignalObject=off  FilterRTWStateStorageClass=Auto  ParallelPVariant=InternalParameters  IdealPVariant=Disabled  IVariant=InternalParameters  DVariant=Disabled  IntegratorVariant=Discrete  SatVariant=Disabled  AWVariant=Passthrough  PCopyVariant=Disabled  TRVariant=Disabled  FdbkBlocksVariant=Forward  IdealPFdbkVariant=Disabled  SatFdbkVariant=Disabled  DerivativeFilterVariant=Disabled  NVariant=Disabled  NCopyVariant=Disabled_SignalSpec  FilterICVariant=Disabled  IntegratorICVariant=InternalICs  ExternalResetVariant=Disabled  TRSumVariant=Passthrough  SumFdbkVariant=Disabled  SumVariant=Sum_PI  TsampFilterVariant=InternalTs  TsampNgainVariant=Passthrough  TsampIntegralVariant=Passthrough  ExternalSaturationOutDataTypeStr=Inherit: Same as second input
  PWM Generator (2-Level) : spsPWMGenerator2LevelLib/PWM Generator (2-Level)  ModulatorType=Three-phase bridge (6 pulses)  ModulatorMode=Unsynchronized  Fc=200*50  Pc=90  nF=27  MinMax="[ -1  1 ]"  SamplingTechnique=Natural  ModulatingSignals=off  m=0.8  Freq=60  Phase=0  Ts=simTs  ShowCarrierOutport=off
  Sum : Sum  Inputs=-+|
  Sum1 : Sum  Inputs=+-|
  Sum2 : Sum  Inputs=++|
  Sum3 : Sum  Inputs=-+|
  Sum4 : Sum  Inputs=--|
  Sum5 : Sum  Inputs=++|
  Vgd1 : InportShadow
  dq0 to abc : spsdq0toabcLib/dq0 to abc  Alignment=90 degrees behind phase A axis
  pwm : Outport
  wires:
  Constant2/1 -> Mux/3
  Gain2/1 -> PWM Generator (2-Level)/1
  Sum1/1 -> Sum2/2
  Sum/1 -> PID Controller/1
  PID Controller/1 -> Sum1/2
  Mux/1 -> dq0 to abc/1
  Sum5/1 -> Mux/2
  dq0 to abc/1 -> Gain2/1
  Gain1/1 -> Sum4/1
  Gain/1 -> Sum1/1
  PID Controller1/1 -> Sum4/2
  Sum3/1 -> PID Controller1/1
  Sum2/1 -> Mux/1
  Sum4/1 -> Sum5/2
  wt/1 -> dq0 to abc/2
  Vgd/1 -> Sum2/1
  Vgq/1 -> Sum5/1
  PWM Generator (2-Level)/1 -> pwm/1
  Gain4/1 -> Divide/1
  Gain5/1 -> Divide1/1
  Pref/1 -> Gain4/1
  Divide/1 -> Sum/2  "Idref"
  Divide1/1 -> Sum3/2  "Iqref"
  Id/1 -> Gain1/1, Sum/1
  Iq/1 -> Gain/1, Sum3/1
  Qref/1 -> Gain5/1
  Vgd1/1 -> IC/1
  IC/1 -> Divide1/2, Divide/2

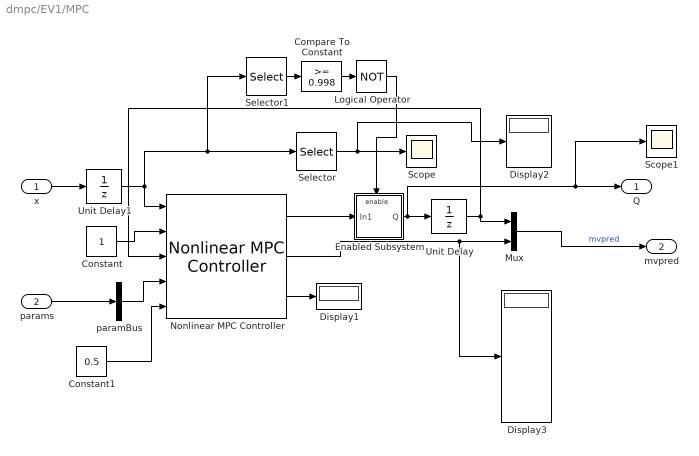
== system dmpc/EV1/MPC ==
  x : Inport
  params : Inport  Port=2
  Compare To Constant : simulink/Logic and Bit Operations/Compare To Constant  relop=>=  const=0.998  OutDataTypeStr=boolean
  Constant : Constant
  Constant1 : Constant  Value=0.5
  Display1 : Display
  Display2 : Display
  Display3 : Display
  Enabled Subsystem : Subsystem  TreatAsAtomicUnit=on
  Logical Operator : Logic  Operator=NOT  AllPortsSameDT=off  OutDataTypeStr=boolean
  Mux : Mux  Inputs=2
  Nonlinear MPC Controller : mpclib/Nonlinear MPC Controller  SCDEnableBlockLinearizationSpecification=on  nlmpcobj=dmpcobj  UseObjectTs=on  UseMEX=off  md_enabled=off  mvtarget_enabled=off  param_enabled=on  cost_enabled=off  mvseq_enabled=on  stateseq_enabled=off  ovseq_enabled=off  slack_enabled=off  status_enabled=on  ov_min=off  ov_max=off  mv_min=off  mv_max=on  mvrate_min=off  mvrate_max=off  state_min=off  state_max=off  ov_weight=off  mv_weight=off  mvrate_weight=off  ecr_weight=off  nlp_initialize=off
  Scope : Scope
  Scope1 : Scope
  Selector : Selector  InputPortWidth=13  IndexOptions=Index vector (dialog)  Indices=[10,11,12]  OutputSizes=1
  Selector1 : Selector  InputPortWidth=13  IndexOptions=Index vector (dialog)  Indices=[10]  OutputSizes=1
  Unit Delay : UnitDelay  InitialCondition=[0]  SampleTime=Ts/2  HasFrameUpgradeWarning=on
  Unit Delay1 : UnitDelay  SampleTime=-1  HasFrameUpgradeWarning=on
  paramBus : BusCreator  Inputs=1  OutDataTypeStr=Bus: paramBus  NonVirtualBus=on
      settings: InheritFromInputs=off
  Q : Outport
  mvpred : Outport  Port=2
  wires:
  Nonlinear MPC Controller/3 -> Display1/1
  x/1 -> Unit Delay1/1
  Unit Delay1/1 -> Nonlinear MPC Controller/1, Selector1/1, Selector/1
  Nonlinear MPC Controller/1 -> Enabled Subsystem/1(In1)
  Constant/1 -> Nonlinear MPC Controller/2
  Selector/1 -> Display2/1, Scope/1
  paramBus/1 -> Nonlinear MPC Controller/4
  Mux/1 -> mvpred/1  "mvpred"
  Unit Delay/1 -> Mux/1, Nonlinear MPC Controller/3
  Nonlinear MPC Controller/2 -> Display3/1, Mux/2
  params/1 -> paramBus/1
  Constant1/1 -> Nonlinear MPC Controller/5
  Enabled Subsystem/1(Q) -> Scope1/1, Q/1, Unit Delay/1
  Selector1/1 -> Compare To Constant/1
  Compare To Constant/1 -> Logical Operator/1
  Logical Operator/1 -> Enabled Subsystem/Enable

== system dmpc/EV1/PLL ==
  Vgq : Inport
  Constant3 : Constant  Value=0
  Display : Display
  Integrator : Integrator
  PID Controller2 : pid_lib/PID Controller  Controller=PI  Form=Parallel  TimeDomain=Continuous-time  UseExternalTs=off  SampleTime=-1  IntegratorMethod=Forward Euler  FilterMethod=Forward Euler  ControllerParametersSource=internal  P=10  I=5000  D=0  UseFilter=on  N=100  TunerSelectOption=Transfer Function Based (PID Tuner App)  InitialConditionSource=internal  InitialConditionForIntegrator=0  InitialConditionForFilter=0  DifferentiatorICPrevScaledInput=0  ExternalReset=none  TrackingMode=off  Kt=1  LimitOutput=off  SatLimitsSource=internal  UpperSaturationLimit=inf  LowerSaturationLimit=-inf  LinearizeAsGain=on  AntiWindupMode=none  Kb=1  POutMin=[]  POutMax=[]  IOutMin=[]  IOutMax=[]  DOutMin=[]  DOutMax=[]  NOutMin=[]  NOutMax=[]  SumOutMin=[]  SumOutMax=[]  SaturationOutMin=[]  SaturationOutMax=[]  PParamMin=[]  PParamMax=[]  IParamMin=[]  IParamMax=[]  DParamMin=[]  DParamMax=[]  NParamMin=[]  NParamMax=[]  KbParamMin=[]  KbParamMax=[]  KtParamMin=[]  KtParamMax=[]  KbOutMin=[]  KbOutMax=[]  KtOutMin=[]  KtOutMax=[]  IntegratorOutMin=[]  IntegratorOutMax=[]  FilterOutMin=[]  FilterOutMax=[]  SumI1OutMin=[]  SumI1OutMax=[]  SumI2OutMin=[]  SumI2OutMax=[]  SumI3OutMin=[]  SumI3OutMax=[]  SumI4OutMin=[]  SumI4OutMax=[]  SumDOutMin=[]  SumDOutMax=[]  DifferentiatorOutMin=[]  DifferentiatorOutMax=[]  FilterDiffOutCoefMin=[]  FilterDiffOutCoefMax=[]  ReciprocalOutMin=[]  ReciprocalOutMax=[]  SumDenOutMin=[]  SumDenOutMax=[]  SumNumOutMin=[]  SumNumOutMax=[]  DivideOutMin=[]  DivideOutMax=[]  UdiffTsProdOutMin=[]  UdiffTsProdOutMax=[]  NTsProdOutMin=[]  NTsProdOutMax=[]  UintegralTsProdOutMin=[]  UintegralTsProdOutMax=[]  UngainTsProdOutMin=[]  UngainTsProdOutMax=[]  IntegratorContinuousStateAttributes=''  IntegratorStateMustResolveToSignalObject=off  IntegratorRTWStateStorageClass=Auto  FilterContinuousStateAttributes=''  FilterStateMustResolveToSignalObject=off  FilterRTWStateStorageClass=Auto  ParallelPVariant=InternalParameters  IdealPVariant=Disabled  IVariant=InternalParameters  DVariant=Disabled  IntegratorVariant=Continuous  SatVariant=Disabled  AWVariant=Passthrough  PCopyVariant=Disabled  TRVariant=Disabled  FdbkBlocksVariant=Forward  IdealPFdbkVariant=Disabled  SatFdbkVariant=Disabled  DerivativeFilterVariant=Disabled  NVariant=Disabled  NCopyVariant=Disabled_SignalSpec  FilterICVariant=Disabled  IntegratorICVariant=InternalICs  ExternalResetVariant=Disabled  TRSumVariant=Passthrough  SumFdbkVariant=Disabled  SumVariant=Sum_PI  TsampFilterVariant=InternalTs  TsampNgainVariant=Passthrough  TsampIntegralVariant=Passthrough  ExternalSaturationOutDataTypeStr=Inherit: Same as second input
  Sum6 : Sum  Inputs=+-|
  wt : Outport
  wires:
  Sum6/1 -> PID Controller2/1
  Integrator/1 -> wt/1
  PID Controller2/1 -> Integrator/1
  Constant3/1 -> Sum6/1
  Vgq/1 -> Display/1, Sum6/2

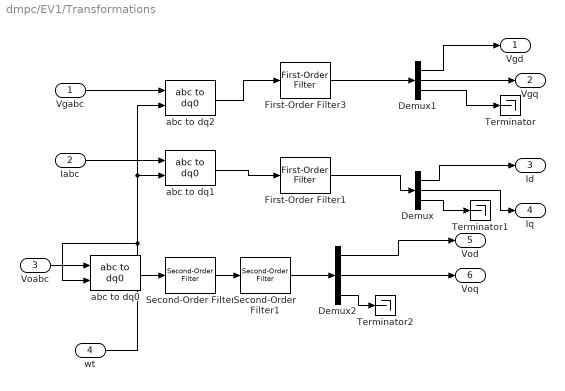
== system dmpc/EV1/Transformations ==
  Vgabc : Inport
  Iabc : Inport  Port=2
  Voabc : Inport  Port=3
  wt : Inport  Port=4
  Demux : Demux  Outputs=3
  Demux1 : Demux  Outputs=3
  Demux2 : Demux  Outputs=3
  First-Order Filter1 : spsFirstOrderFilterLib/First-Order Filter  FilterType=Lowpass  Tc=150e-6  Ts=0  Initialize=off  Vac_Init=[0, 0, 50]  Vdc_Init=0  PlotResponse=off  FreqRange="[0,  200,  1]"
  First-Order Filter3 : spsFirstOrderFilterLib/First-Order Filter  FilterType=Lowpass  Tc=150e-6  Ts=0  Initialize=off  Vac_Init=[0, 0, 50]  Vdc_Init=0  PlotResponse=off  FreqRange="[0,  200,  1]"
  Second-Order Filter : spsSecondOrderFilterLib/Second-Order Filter  FilterType=Lowpass  Fo=1000  Zeta=0.8  Ts=0  Initialize=off  Vac_Init="[0,  0,  60]"  Vdc_Init=0  PlotResponse=off  FreqRange=[0, 10000, 10]
      settings: SourceProductBaseCode=PS
  Second-Order Filter1 : spsSecondOrderFilterLib/Second-Order Filter  FilterType=Lowpass  Fo=1000  Zeta=0.8  Ts=0  Initialize=off  Vac_Init="[0,  0,  60]"  Vdc_Init=0  PlotResponse=off  FreqRange=[0, 10000, 10]
      settings: SourceProductBaseCode=PS
  Terminator : Terminator
  Terminator1 : Terminator
  Terminator2 : Terminator
  abc to dq0 : spsabctodq0Lib/abc to dq0  Alignment=90 degrees behind phase A axis
  abc to dq1 : spsabctodq0Lib/abc to dq0  Alignment=90 degrees behind phase A axis
  abc to dq2 : spsabctodq0Lib/abc to dq0  Alignment=90 degrees behind phase A axis
  Vgd : Outport
  Vgq : Outport  Port=2
  Id : Outport  Port=3
  Iq : Outport  Port=4
  Vod : Outport  Port=5
  Voq : Outport  Port=6
  wires:
  abc to dq2/1 -> First-Order Filter3/1
  abc to dq1/1 -> First-Order Filter1/1
  Demux/3 -> Terminator1/1
  Demux1/1 -> Vgd/1
  Vgabc/1 -> abc to dq2/1
  Demux/1 -> Id/1
  Demux1/2 -> Vgq/1
  Demux/2 -> Iq/1
  Demux1/3 -> Terminator/1
  Iabc/1 -> abc to dq1/1
  Demux2/2 -> Voq/1
  Second-Order Filter1/1 -> Demux2/1
  Demux2/1 -> Vod/1
  Second-Order Filter/1 -> Second-Order Filter1/1
  wt/1 -> abc to dq2/2, abc to dq1/2, abc to dq0/2
  Voabc/1 -> abc to dq0/1
  abc to dq0/1 -> Second-Order Filter/1
  Demux2/3 -> Terminator2/1
  First-Order Filter3/1 -> Demux1/1
  First-Order Filter1/1 -> Demux/1

== system dmpc/EV2/Bus Voltage Measurement ==
  Vgabc : Inport
  Bus Creator : BusCreator  Inputs=2
  Demux : Demux  Outputs=3
  Fourier1 : spsFourierLib/Fourier  Freq=50  n=1  InInit=[300, 0]  Ts=simTs
      settings: SourceProductBaseCode=PS
  Gain : Gain  Gain=sqrt(3/2)/400
  Gain1 : Gain  Gain=pi/180
  Scope : Scope
  Terminator : Terminator
  Terminator1 : Terminator
  Bus Voltage : Outport
  wires:
  Gain/1 -> Bus Creator/2  "voltage"
  Bus Creator/1 -> Bus Voltage/1
  Fourier1/1 -> Gain/1
  Demux/1 -> Fourier1/1
  Vgabc/1 -> Demux/1
  Gain1/1 -> Scope/1, Bus Creator/1  "theta"
  Fourier1/2 -> Gain1/1
  Demux/2 -> Terminator/1
  Demux/3 -> Terminator1/1
